simulink model "zadamie1"  (R2025b)
settings: Solver=VariableStepAuto  StartTime=0.0  StopTime=0.1  RelTol=1e-3
values from neighbouring files (symbols this model uses):
  B = 0.00981    [CV1.m]
  Cu = 4.86    [CV1.m]
  J = 0.004    [CV1.m]
  L = 156.2 * 10^-3    (= 0.1562)    [CV1.m]
  R = 54.38    [CV1.m]
settings Model: Creator=jakub  LastModifiedBy=jakub

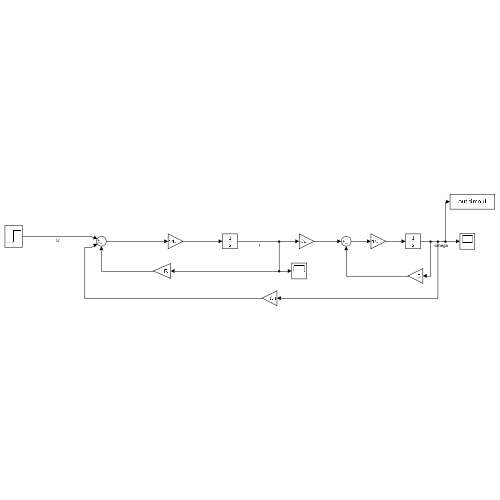
[thumbnail: Simulink's stored preview of the top-level diagram]
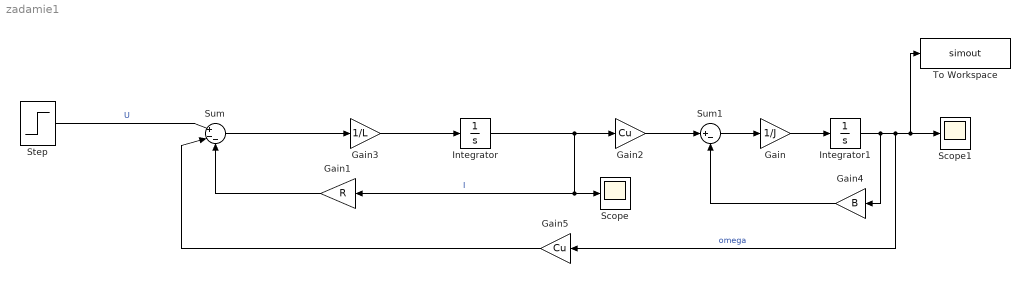
== system zadamie1 ==
  Gain : Gain  Gain=1/J
  Gain1 : Gain  Gain=R
  Gain2 : Gain  Gain=Cu
  Gain3 : Gain  Gain=1/L
  Gain4 : Gain  Gain=B
  Gain5 : Gain  Gain=Cu
  Integrator : Integrator
  Integrator1 : Integrator
  Scope : Scope
      settings: ActiveDisplayYMinimum=-0.36693292601182631  ActiveDisplayYMaximum=0.76443596443660433
  Scope1 : Scope
      settings: ActiveDisplayYMinimum=52.438935466827289  ActiveDisplayYMaximum=57.754931559261706
  Step : Step  Time=0.05  After=280  SampleTime=0
  Sum : Sum  Inputs=|+--
  Sum1 : Sum  Inputs=|+-
  To Workspace : ToWorkspace  VariableName=simout  SaveFormat=Timeseries  SampleTime=-1
  wires:
  Step/1 -> Sum/1  "U"
  Sum/1 -> Gain3/1
  Gain3/1 -> Integrator/1
  Integrator/1 -> Gain2/1, Gain1/1, Scope/1  "I"
  Gain1/1 -> Sum/3
  Gain2/1 -> Sum1/1
  Sum1/1 -> Gain/1
  Gain/1 -> Integrator1/1
  Gain4/1 -> Sum1/2
  Integrator1/1 -> Gain5/1, To Workspace/1, Scope1/1, Gain4/1  "omega"
  Gain5/1 -> Sum/2
